simulink model "CombinedExperiment"  (R2020a)
settings: Solver=FixedStepAuto  StartTime=0.0  StopTime=tsim  FixedStep=baseRate  RelTol=1e-3  EnableMultiTasking=on
values from neighbouring files (symbols this model uses):
  baseRate = 1/10    (= 0.1)    [Run_Initializer.m]
  drop_states_BLACK = [ 0.6; 0.6; target_starting_angle]    [Run_Initializer.m]
  drop_states_BLUE = [ xLength/2+0.9; yLength/2+0.5; 0]    [Run_Initializer.m]
  drop_states_RED = [ xLength/2+0.6; yLength/2; pi]    [Run_Initializer.m]
  F_thrusters_BLACK = 0.25.*ones(8,1)    [Run_Initializer.m]
  F_thrusters_BLUE = 0.25.*ones(8,1)    [Run_Initializer.m]
  F_thrusters_RED = 0.25.*ones(8,1)    [Run_Initializer.m]
  home_states_BLACK = [ 0.6; 0.6; target_starting_angle]    [Run_Initializer.m]
  home_states_BLUE = [ xLength/2-0.9; yLength/2+0.5; 0]    [Run_Initializer.m]
  home_states_RED = [ xLength/2+0.6; yLength/2; pi]    [Run_Initializer.m]
  init_states_BLACK = [ 0.6; 0.6; target_starting_angle]    [Run_Initializer.m]
  init_states_BLUE = [ xLength/2+0.9; yLength/2+0.5; 0]    [Run_Initializer.m]
  init_states_RED = [ xLength/2+0.6; yLength/2; pi]    [Run_Initializer.m]
  Kd_tb = 0.4/5    (= 0.08)    [Run_Initializer.m]
  Kd_tblue = 0.4    [Run_Initializer.m]
  Kd_tr = 0.4    [Run_Initializer.m]
  Kd_xb = 5    [Run_Initializer.m]
  Kd_xblue = 5    [Run_Initializer.m]
  Kd_xr = 5    [Run_Initializer.m]
  Kd_yb = 5    [Run_Initializer.m]
  Kd_yblue = 5    [Run_Initializer.m]
  Kd_yr = 5    [Run_Initializer.m]
  Kp_tb = 0.1/5    (= 0.02)    [Run_Initializer.m]
  Kp_tblue = 0.1    [Run_Initializer.m]
  Kp_tr = 0.1    [Run_Initializer.m]
  Kp_xb = 2    [Run_Initializer.m]
  Kp_xblue = 2    [Run_Initializer.m]
  Kp_xr = 2    [Run_Initializer.m]
  Kp_yb = 2    [Run_Initializer.m]
  Kp_yblue = 2    [Run_Initializer.m]
  Kp_yr = 2    [Run_Initializer.m]
  noise_variance_BLACK = 0    [Run_Initializer.m]
  noise_variance_BLUE = 0    [Run_Initializer.m]
  noise_variance_RED = 0    [Run_Initializer.m]
  Phase0_End = Phase0_Duration    (= 8)    [Run_Initializer.m]
  Phase1_End = Phase0_Duration + Phase1_Duration    (= 13)    [Run_Initializer.m]
  Phase2_End = Phase0_Duration + Phase1_Duration +                                   Phase2_Duration    (= 38)    [Run_Initializer.m]
  Phase3_End = Phase0_Duration + Phase1_Duration +                                   Phase2_Duration + Phase3_Duration    (= 215)    [Run_Initializer.m]
  Phase3_SubPhase1_End = Phase2_End + Phase3_SubPhase1_Duration    (= 41)    [Run_Initializer.m]
  Phase3_SubPhase2_End = Phase2_End + Phase3_SubPhase1_Duration +                                   Phase3_SubPhase2_Duration    (= 42)    [Run_Initializer.m]
  Phase3_SubPhase3_End = Phase2_End + Phase3_SubPhase1_Duration +                                   Phase3_SubPhase2_Duration +                                  Phase3_SubPhase3_Duration    (= 72)    [Run_Initializer.m]
  Phase3_SubPhase4_End = Phase2_End + Phase3_SubPhase1_Duration +                                   Phase3_SubPhase2_Duration +                                  Phase3_SubPhase3_Duration +                                  Phase3_SubPhase4_Duration    [Run_Initializer.m]
  Phase4_End = Phase0_Duration + Phase1_Duration +                                   Phase2_Duration + Phase3_Duration +                                   Phase4_Duration    (= 235)    [Run_Initializer.m]
  Phase5_End = Phase0_Duration + Phase1_Duration +                                   Phase2_Duration + Phase3_Duration +                                   Phase4_Duration + Phase5_Duration    (= 240)    [Run_Initializer.m]
  serverRate = 1/5    (= 0.2)    [Run_Initializer.m]
  target_angular_velocity = 0.1    [Run_Initializer.m]
  thruster_dist2CG_BLACK = [83.42;-52.58;55.94;-60.05;54.08;-53.92;77.06;-55.94]    [Run_Initializer.m]
  thruster_dist2CG_BLUE = [83.42;-52.58;55.94;-60.05;54.08;-53.92;77.06;-55.94]    [Run_Initializer.m]
  thruster_dist2CG_RED = [49.92;-78.08;70.46;-63.54;81.08;-50.42;57.44;-75.96]    [Run_Initializer.m]
undefined symbols (not defined in the file or in its folder): DiscIntNeverNeededParam, platformSelection, simMode, WhoAmI
libraries: dspstat3 x18, dspsigops x12, raspberrypiBasiclib x10, embdlinuxlib x8, simulink x8, MainLibrary x6, mspfiltlib x3, dsparch4 x3, dspswit3 x2, sensehatlib x1
(part 5 of 10)

== system CombinedExperiment/Phase #3: Experiment/Change RED Behavior/Sub-Phase #3  ==
  note: ARM Control Law - RED
  note: PD Control Law - RED
  note: Additional Blocks
  note: Additional blocks are stored above. Note that to control attitude using the RW, simply replace RED_Tz with RED_Tz_RW.
  note: This section is reserved for any control law for the robotic manipulator.
  Action Port : ActionPort  ActionPortLabel=elseif( u1 < u4)
  1-D Lookup Table : Lookup_n-D  NumberOfTableDimensions=1  BreakpointsForDimension1=|  Table=|  InternalRulePriority=Speed  RndMeth=Simplest  InputSameDT=on
      BreakpointsForDimension1=|
      | [42
      | 42.01112133
      | 42.03727126
      | 42.07834039
      | 42.13428459
      | 42.20504754
      | 42.29055854
      | 42.39073228
      | 42.5054689
      | 42.63465399
      | 42.77815879
      | 42.93584024
      | 43.10754115
      | 43.29309037
      | 43.49230294
      | 43.70498028
      | 43.93091039
      | 44.16986804
      | 44.42161506
      | 44.68590048
      | 44.96246087
      | 45.25102053
      | 45.55129184
      | 45.86297547
      | 46.18576072
      | 46.51932585
      | 46.86333834
      | 47.21745527
      | 47.58132366
      | 47.95458079
      | 48.33685459
      | 48.727764
      | 49.12691936
      | 49.53392277
      | 49.94836853
      | 50.36984352
      | 50.79792758
      | 51.23219401
      | 51.67220991
      | 52.11753667
      | 52.56773038
      | 53.02234226
      | 53.48091917
      | 53.94300397
      | 54.40813605
      | 54.87585175
      | 55.34568486
      | 55.81716702
      | 56.28982825
      | 56.7631974
      | 57.2368026
      | 57.71017175
      | 58.18283298
      | 58.65431514
      | 59.12414825
      | 59.59186395
      | 60.05699603
      | 60.51908083
      | 60.97765774
      | 61.43226962
      | 61.88246333
      | 62.32779009
      | 62.76780599
      | 63.20207242
      | 63.63015648
      | 64.05163147
      | 64.46607723
      | 64.87308064
      | 65.272236
      | 65.66314541
      | 66.04541921
      | 66.41867634
      | 66.78254473
      | 67.13666166
      | 67.48067415
      | 67.81423928
      | 68.13702453
      | 68.44870816
      | 68.74897947
      | 69.03753913
      | 69.31409952
      | 69.57838494
      | 69.83013196
      | 70.06908961
      | 70.29501972
      | 70.50769706
      | 70.70690963
      | 70.89245885
      | 71.06415976
      | 71.22184121
      | 71.36534601
      | 71.4945311
      | 71.60926772
      | 71.70944146
      | 71.79495246
      | 71.86571541
      | 71.92165961
      | 71.96272874
      | 71.98887867
      | 72
      | ]
      Table=|
      | [1.570796327
      | 1.570792957
      | 1.570647694
      | 1.56961565
      | 1.567632601
      | 1.56219496
      | 1.557494298
      | 1.549269077
      | 1.544187815
      | 1.533149542
      | 1.522693414
      | 1.496131515
      | 1.446175572
      | 1.373291416
      | 1.270392573
      | 1.167493418
      | 1.052460989
      | 0.935207834
      | 0.807889258
      | 0.677163853
      | 0.538528963
      | 0.394913096
      | 0.249656169
      | 0.099916299
      | -0.053813644
      | -0.205103655
      | -0.380299244
      | -0.546735993
      | -0.717860815
      | -0.811444171
      | -0.923417052
      | -0.9559831
      | -0.833382367
      | -0.653115778
      | -0.440627342
      | -0.233135617
      | -0.016770488
      | 0.198541763
      | 0.420037648
      | 0.64133109
      | 0.8678487
      | 1.093144441
      | 1.326954733
      | 1.513077918
      | 1.568710242
      | 1.570730531
      | 1.567250769
      | 1.570752371
      | 1.57074092
      | 1.549011834
      | 1.401751602
      | 1.165146113
      | 1.0076873
      | 0.810904438
      | 0.65519077
      | 0.460795111
      | 0.26479445
      | 0.068785172
      | -0.154928236
      | -0.361424338
      | -0.588740331
      | -0.797757514
      | -1.025114417
      | -1.236311075
      | -1.435945334
      | -1.511406602
      | -1.466017975
      | -1.310813705
      | -1.105992736
      | -0.913718388
      | -0.722685301
      | -0.536202121
      | -0.354350457
      | -0.177037457
      | -0.005416103
      | 0.161859666
      | 0.322652337
      | 0.479244088
      | 0.627815916
      | 0.771700562
      | 0.909552257
      | 1.042365309
      | 1.164760086
      | 1.265366299
      | 1.329745445
      | 1.358265779
      | 1.355564401
      | 1.328554047
      | 1.279612684
      | 1.24723853
      | 1.197192467
      | 1.141005155
      | 1.106426692
      | 1.08119376
      | 1.067581158
      | 1.058578831
      | 1.055001377
      | 1.05322972
      | 1.052803704
      | 1.052721605
      | ]
  1-D Lookup Table1 : Lookup_n-D  NumberOfTableDimensions=1  BreakpointsForDimension1=|  Table=|  InternalRulePriority=Speed  RndMeth=Simplest  InputSameDT=on
      BreakpointsForDimension1=|
      | [42
      | 42.01112133
      | 42.03727126
      | 42.07834039
      | 42.13428459
      | 42.20504754
      | 42.29055854
      | 42.39073228
      | 42.5054689
      | 42.63465399
      | 42.77815879
      | 42.93584024
      | 43.10754115
      | 43.29309037
      | 43.49230294
      | 43.70498028
      | 43.93091039
      | 44.16986804
      | 44.42161506
      | 44.68590048
      | 44.96246087
      | 45.25102053
      | 45.55129184
      | 45.86297547
      | 46.18576072
      | 46.51932585
      | 46.86333834
      | 47.21745527
      | 47.58132366
      | 47.95458079
      | 48.33685459
      | 48.727764
      | 49.12691936
      | 49.53392277
      | 49.94836853
      | 50.36984352
      | 50.79792758
      | 51.23219401
      | 51.67220991
      | 52.11753667
      | 52.56773038
      | 53.02234226
      | 53.48091917
      | 53.94300397
      | 54.40813605
      | 54.87585175
      | 55.34568486
      | 55.81716702
      | 56.28982825
      | 56.7631974
      | 57.2368026
      | 57.71017175
      | 58.18283298
      | 58.65431514
      | 59.12414825
      | 59.59186395
      | 60.05699603
      | 60.51908083
      | 60.97765774
      | 61.43226962
      | 61.88246333
      | 62.32779009
      | 62.76780599
      | 63.20207242
      | 63.63015648
      | 64.05163147
      | 64.46607723
      | 64.87308064
      | 65.272236
      | 65.66314541
      | 66.04541921
      | 66.41867634
      | 66.78254473
      | 67.13666166
      | 67.48067415
      | 67.81423928
      | 68.13702453
      | 68.44870816
      | 68.74897947
      | 69.03753913
      | 69.31409952
      | 69.57838494
      | 69.83013196
      | 70.06908961
      | 70.29501972
      | 70.50769706
      | 70.70690963
      | 70.89245885
      | 71.06415976
      | 71.22184121
      | 71.36534601
      | 71.4945311
      | 71.60926772
      | 71.70944146
      | 71.79495246
      | 71.86571541
      | 71.92165961
      | 71.96272874
      | 71.98887867
      | 72
      | ]
      Table=|
      | [1.57079632679490
      | 1.57079662136271
      | 1.57035858393418
      | 1.56955473957150
      | 1.56795883023701
      | 1.56855196252543
      | 1.56956191136717
      | 1.57072970527338
      | 1.57079005485722
      | 1.56948791223666
      | 1.55119006552306
      | 1.55836585845583
      | 1.57077777185491
      | 1.57077149370545
      | 1.57076310797240
      | 1.57036928804412
      | 1.57074947684855
      | 1.56898331366692
      | 1.57073740451593
      | 1.56257826917437
      | 1.57072974696569
      | 1.56230742665956
      | 1.57073312881541
      | 1.56360724537446
      | 1.57075185491036
      | 1.56920954766940
      | 1.57077382899638
      | 1.54477346684241
      | 1.38400507014983
      | 1.23109269186081
      | 1.02321737126326
      | 0.866665055111140
      | 0.663320579242585
      | 0.523334911886864
      | 0.348534652658928
      | 0.228481728516264
      | 0.156644623807384
      | 0.0854385589397119
      | 0.0684187356026291
      | -0.0143597952556130
      | -0.0517524216410004
      | -0.0928804549026143
      | -0.215704480084781
      | -0.422252680325216
      | -0.607845118006062
      | -0.846263996013364
      | -1.04958098308095
      | -1.27739473865326
      | -1.42310649047080
      | -1.57075277736191
      | -1.57072459354704
      | -1.57072993276777
      | -1.54331811766860
      | -1.57073414073308
      | -1.55931623516956
      | -1.57073842553777
      | -1.57072399077284
      | -1.57072720156105
      | -1.57071264380253
      | -1.56934197452670
      | -1.57070564382063
      | -1.56141817042798
      | -1.57070830688086
      | -1.49469854852628
      | -1.31259934378585
      | -1.11020895684375
      | -0.916078821647610
      | -0.731793274192232
      | -0.573229556030265
      | -0.475634259727501
      | -0.252113034776861
      | -0.175932768714599
      | -0.117451385657779
      | -0.113075584941122
      | -0.108548532723191
      | -0.120323450723243
      | -0.116071199535664
      | -0.122092030089114
      | -0.179069682787195
      | -0.187679506880811
      | -0.283142131452161
      | -0.409036068532655
      | -0.536944980678811
      | -0.655297933993903
      | -0.768540738868273
      | -0.875433002578302
      | -0.973536605110186
      | -1.06911393555782
      | -1.14791786909907
      | -1.22902449271238
      | -1.27006052589809
      | -1.28669314276116
      | -1.31617501989999
      | -1.33099075176741
      | -1.34662299508091
      | -1.35249457213426
      | -1.35797341773929
      | -1.35939252934314
      | -1.35990006404006
      | -1.35985448160842]
  1-D Lookup Table2 : Lookup_n-D  NumberOfTableDimensions=1  BreakpointsForDimension1=|  Table=|  InternalRulePriority=Speed  RndMeth=Simplest  InputSameDT=on
      BreakpointsForDimension1=|
      | [42
      | 42.01112133
      | 42.03727126
      | 42.07834039
      | 42.13428459
      | 42.20504754
      | 42.29055854
      | 42.39073228
      | 42.5054689
      | 42.63465399
      | 42.77815879
      | 42.93584024
      | 43.10754115
      | 43.29309037
      | 43.49230294
      | 43.70498028
      | 43.93091039
      | 44.16986804
      | 44.42161506
      | 44.68590048
      | 44.96246087
      | 45.25102053
      | 45.55129184
      | 45.86297547
      | 46.18576072
      | 46.51932585
      | 46.86333834
      | 47.21745527
      | 47.58132366
      | 47.95458079
      | 48.33685459
      | 48.727764
      | 49.12691936
      | 49.53392277
      | 49.94836853
      | 50.36984352
      | 50.79792758
      | 51.23219401
      | 51.67220991
      | 52.11753667
      | 52.56773038
      | 53.02234226
      | 53.48091917
      | 53.94300397
      | 54.40813605
      | 54.87585175
      | 55.34568486
      | 55.81716702
      | 56.28982825
      | 56.7631974
      | 57.2368026
      | 57.71017175
      | 58.18283298
      | 58.65431514
      | 59.12414825
      | 59.59186395
      | 60.05699603
      | 60.51908083
      | 60.97765774
      | 61.43226962
      | 61.88246333
      | 62.32779009
      | 62.76780599
      | 63.20207242
      | 63.63015648
      | 64.05163147
      | 64.46607723
      | 64.87308064
      | 65.272236
      | 65.66314541
      | 66.04541921
      | 66.41867634
      | 66.78254473
      | 67.13666166
      | 67.48067415
      | 67.81423928
      | 68.13702453
      | 68.44870816
      | 68.74897947
      | 69.03753913
      | 69.31409952
      | 69.57838494
      | 69.83013196
      | 70.06908961
      | 70.29501972
      | 70.50769706
      | 70.70690963
      | 70.89245885
      | 71.06415976
      | 71.22184121
      | 71.36534601
      | 71.4945311
      | 71.60926772
      | 71.70944146
      | 71.79495246
      | 71.86571541
      | 71.92165961
      | 71.96272874
      | 71.98887867
      | 72
      | ]
      Table=|
      | [-1.10360555189321e-17
      | -0.000682555954124297
      | -0.000504375242443253
      | 0.00336297359381415
      | 0.0137095670724727
      | 0.0252677971790659
      | 0.0446557220510096
      | 0.0672113326003172
      | 0.0999781977666613
      | 0.137287456967193
      | 0.189071248486376
      | 0.272294508037825
      | 0.355665679231944
      | 0.446845913729827
      | 0.544137284526667
      | 0.639346413276106
      | 0.732541458867562
      | 0.808938354869002
      | 0.855848674103189
      | 0.891616122311551
      | 0.876064789878543
      | 0.835218274860764
      | 0.735847487773707
      | 0.623237833236767
      | 0.450912596118759
      | 0.313068707480842
      | 0.118982751928026
      | -0.0346963999777990
      | -0.244244268013732
      | -0.386045753956551
      | -0.607135995230889
      | -0.645065479955685
      | -0.658232101032023
      | -0.707283001569499
      | -0.727739337943063
      | -0.773334139757485
      | -0.790813868197939
      | -0.829315581367480
      | -0.831591865361474
      | -0.895741116707505
      | -0.917692198886409
      | -0.966835773186509
      | -1.05732301030663
      | -1.15418729750044
      | -1.28905944926691
      | -1.41505461173534
      | -1.40486598987903
      | -1.38850533888304
      | -1.31148648974968
      | -1.22739644537344
      | -1.09679708257291
      | -1.01375741649069
      | -0.900389419892854
      | -0.817697106109663
      | -0.706296706872995
      | -0.627649901158471
      | -0.522783214749143
      | -0.449254069405809
      | -0.350308226521183
      | -0.271181857633944
      | -0.185730374564875
      | -0.134238582279295
      | -0.0589333568892688
      | -0.0193632216828676
      | 0.0500980441953301
      | 0.0783818433368992
      | 0.203392718385905
      | 0.287418813233287
      | 0.286916152215522
      | 0.228277773431529
      | 0.205391483508272
      | 0.153166933412198
      | 4.01249706205260e-05
      | -0.106583281044124
      | -0.214939176631723
      | -0.275105513577021
      | -0.328996825397653
      | -0.353637536054736
      | -0.366278937268333
      | -0.349072653017436
      | -0.324125317636826
      | -0.291582405014021
      | -0.240949835499918
      | -0.195848531903513
      | -0.143488080387155
      | -0.0988801304986467
      | -0.0443831356850743
      | 0.00807376276159867
      | 0.0766461923527033
      | 0.116804310925055
      | 0.159885004199221
      | 0.212747759359235
      | 0.240304582731963
      | 0.265011768867661
      | 0.280740585503698
      | 0.294154580752225
      | 0.300980006322197
      | 0.305531467486406
      | 0.306822115333088
      | 0.307132876918720]
  Constant{,1,4..6} (5 alike) : Constant  Value=0
  Data Store Read : DataStoreRead  DataStoreName=Univ_Time
  Data Store Write : DataStoreWrite  DataStoreName=RED_Tz_Shoulder
  Data Store Write1 : DataStoreWrite  DataStoreName=RED_Tz_Elbow
  Data Store Write2 : DataStoreWrite  DataStoreName=RED_Tz_Wrist
  Data Store Write3 : DataStoreWrite  DataStoreName=Float_State
  From Workspace : FromWorkspace  Commented=on  VariableName=Pos_J1  SampleTime=-1
  From Workspace1 : FromWorkspace  Commented=on  VariableName=Pos_J2  SampleTime=-1
  From Workspace2 : FromWorkspace  Commented=on  VariableName=Pos_J3  SampleTime=-1
  Puck State : Constant
  RED_Fx : DataStoreWrite  DataStoreName=RED_Fx
  RED_Fy : DataStoreWrite  DataStoreName=RED_Fy
  RED_Tz : DataStoreWrite  DataStoreName=RED_Tz
  RED_Tz_RW : DataStoreWrite  DataStoreName=RED_Tz_RW
  Send Position Commands to Manipulator : MainLibrary/Dynamixel Functions/Send Position Commands to Manipulator  Commented=on
      settings: SourceProductName=SPOT Custom Library
  Send Position Commands to Manipulator1 : MainLibrary/Dynamixel Functions/Send Position Commands to Manipulator
      settings: SourceProductName=SPOT Custom Library
  wires:
  Constant1/1 -> RED_Tz_RW/1
  Constant6/1 -> Data Store Write2/1
  Constant4/1 -> Data Store Write/1
  Constant5/1 -> Data Store Write1/1
  Constant/1 -> RED_Tz/1, RED_Fx/1, RED_Fy/1
  Puck State/1 -> Data Store Write3/1
  From Workspace2/1 -> Send Position Commands to Manipulator/3
  From Workspace1/1 -> Send Position Commands to Manipulator/2
  From Workspace/1 -> Send Position Commands to Manipulator/1
  1-D Lookup Table2/1 -> Send Position Commands to Manipulator1/3
  Data Store Read/1 -> 1-D Lookup Table2/1, 1-D Lookup Table1/1, 1-D Lookup Table/1
  1-D Lookup Table1/1 -> Send Position Commands to Manipulator1/2
  1-D Lookup Table/1 -> Send Position Commands to Manipulator1/1

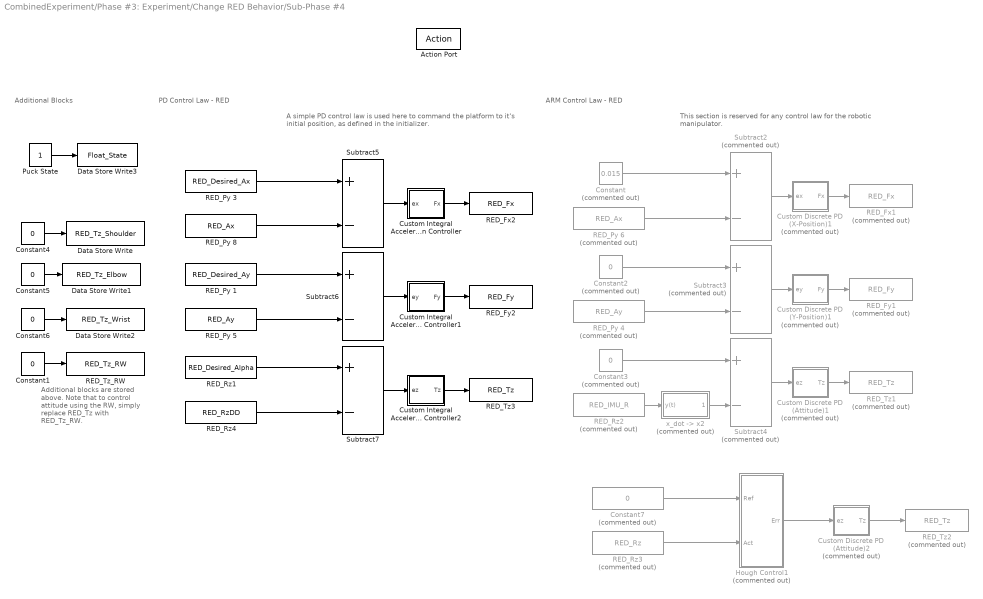
== system CombinedExperiment/Phase #3: Experiment/Change RED Behavior/Sub-Phase #4 ==
  note: ARM Control Law - RED
  note: PD Control Law - RED
  note: Additional Blocks
  note: Additional blocks are stored above. Note that to control attitude using the RW, simply replace RED_Tz with RED_Tz_RW.
  note: A simple PD control law is used here to command the platform to it's initial position, as defined in the initializer.
  note: This section is reserved for any control law for the robotic manipulator.
  Action Port : ActionPort  ActionPortLabel=elseif( u1 < u5)
  Constant : Constant  Commented=on  Value=0.015
  Constant{1,4..6} (4 alike) : Constant  Value=0
  Constant2 : Constant  Commented=on  Value=0
  Constant3 : Constant  Commented=on  Value=0
  Constant7 : Constant  Commented=on  Value=0
  Custom Discrete PD (Attitude)1 : Subsystem  Commented=on
  Custom Discrete PD (Attitude)2 : Subsystem  Commented=on
  Custom Discrete PD (X-Position)1 : Subsystem  Commented=on
  Custom Discrete PD (Y-Position)1 : Subsystem  Commented=on
  Custom Integral Acceleration Controller : Subsystem
  Custom Integral Acceleration Controller1 : Subsystem
  Custom Integral Acceleration Controller2 : Subsystem
  Data Store Write : DataStoreWrite  DataStoreName=RED_Tz_Shoulder
  Data Store Write1 : DataStoreWrite  DataStoreName=RED_Tz_Elbow
  Data Store Write2 : DataStoreWrite  DataStoreName=RED_Tz_Wrist
  Data Store Write3 : DataStoreWrite  DataStoreName=Float_State
  Hough Control1 : Subsystem  Commented=on
  Puck State : Constant
  RED_Fx1 : DataStoreWrite  Commented=on  DataStoreName=RED_Fx
  RED_Fx2 : DataStoreWrite  DataStoreName=RED_Fx
  RED_Fy1 : DataStoreWrite  Commented=on  DataStoreName=RED_Fy
  RED_Fy2 : DataStoreWrite  DataStoreName=RED_Fy
  RED_Py 1 : DataStoreRead  DataStoreName=RED_Desired_Ay
  RED_Py 3 : DataStoreRead  DataStoreName=RED_Desired_Ax
  RED_Py 4 : DataStoreRead  Commented=on  DataStoreName=RED_Ay
  RED_Py 5 : DataStoreRead  DataStoreName=RED_Ay
  RED_Py 6 : DataStoreRead  Commented=on  DataStoreName=RED_Ax
  RED_Py 8 : DataStoreRead  DataStoreName=RED_Ax
  RED_Rz1 : DataStoreRead  DataStoreName=RED_Desired_Alpha
  RED_Rz2 : DataStoreRead  Commented=on  DataStoreName=RED_IMU_R
  RED_Rz3 : DataStoreRead  Commented=on  DataStoreName=RED_Rz
  RED_Rz4 : DataStoreRead  DataStoreName=RED_RzDD
  RED_Tz1 : DataStoreWrite  Commented=on  DataStoreName=RED_Tz
  RED_Tz2 : DataStoreWrite  Commented=on  DataStoreName=RED_Tz
  RED_Tz3 : DataStoreWrite  DataStoreName=RED_Tz
  RED_Tz_RW : DataStoreWrite  DataStoreName=RED_Tz_RW
  Subtract2 : Sum  Commented=on  Inputs=+-
  Subtract3 : Sum  Commented=on  Inputs=+-
  Subtract4 : Sum  Commented=on  Inputs=+-
  Subtract5 : Sum  Inputs=+-
  Subtract6 : Sum  Inputs=+-
  Subtract7 : Sum  Inputs=+-
  "x_dot -> x2" : Subsystem  Commented=on
  wires:
  Constant1/1 -> RED_Tz_RW/1
  Constant6/1 -> Data Store Write2/1
  Constant4/1 -> Data Store Write/1
  Constant5/1 -> Data Store Write1/1
  Puck State/1 -> Data Store Write3/1
  Constant2/1 -> Subtract3/1
  "x_dot -> x2"/1(dy(t)/dt) -> Subtract4/2
  Subtract3/1 -> Custom Discrete PD (Y-Position)1/1(ey)
  Constant3/1 -> Subtract4/1
  RED_Py 4/1 -> Subtract3/2
  RED_Rz2/1 -> "x_dot -> x2"/1(y(t))
  Custom Discrete PD (Attitude)1/1(Tz) -> RED_Tz1/1
  RED_Py 6/1 -> Subtract2/2
  Subtract2/1 -> Custom Discrete PD (X-Position)1/1(ex)
  Custom Discrete PD (X-Position)1/1(Fx) -> RED_Fx1/1
  Subtract4/1 -> Custom Discrete PD (Attitude)1/1(ez)
  Constant/1 -> Subtract2/1
  Custom Discrete PD (Y-Position)1/1(Fy) -> RED_Fy1/1
  Hough Control1/1(Err) -> Custom Discrete PD (Attitude)2/1(ez)
  Constant7/1 -> Hough Control1/1(Ref)
  RED_Rz3/1 -> Hough Control1/2(Act)
  Custom Discrete PD (Attitude)2/1(Tz) -> RED_Tz2/1
  Subtract6/1 -> Custom Integral Acceleration Controller1/1(ey)
  Subtract5/1 -> Custom Integral Acceleration Controller/1(ex)
  RED_Py 8/1 -> Subtract5/2
  RED_Rz4/1 -> Subtract7/2
  Subtract7/1 -> Custom Integral Acceleration Controller2/1(ez)
  RED_Py 5/1 -> Subtract6/2
  Custom Integral Acceleration Controller2/1(Tz) -> RED_Tz3/1
  Custom Integral Acceleration Controller1/1(Fy) -> RED_Fy2/1
  Custom Integral Acceleration Controller/1(Fx) -> RED_Fx2/1
  RED_Py 3/1 -> Subtract5/1
  RED_Py 1/1 -> Subtract6/1
  RED_Rz1/1 -> Subtract7/1

== system CombinedExperiment/Phase #3: Experiment/Change RED Behavior/Subsystem ==
  Universal_Time : DataStoreRead  DataStoreName=Univ_Time
  Time : Outport  VectorParamsAs1DForOutWhenUnconnected=off
  wires:
  Universal_Time/1 -> Time/1

== system CombinedExperiment/Phase #4: Return Home/Change BLACK Behavior/Custom Discrete PD (Attitude) ==
  ez : Inport
  Sum3 : Sum
  kd_tb : Gain  Gain=Kd_tb
  kp_tb : Gain  Gain=Kp_tb
  "x_dot -> x1" : Subsystem
  Tz : Outport  VectorParamsAs1DForOutWhenUnconnected=off
  wires:
  kd_tb/1 -> Sum3/1
  Sum3/1 -> Tz/1
  kp_tb/1 -> Sum3/2
  "x_dot -> x1"/1(dy(t)/dt) -> kd_tb/1
  ez/1 -> "x_dot -> x1"/1(y(t)), kp_tb/1

== system CombinedExperiment/Phase #4: Return Home/Change BLACK Behavior/Custom Discrete PD (X-Position) ==
  ex : Inport
  Sum3 : Sum
  kd_xb : Gain  Gain=Kd_xb
  kp_xb : Gain  Gain=Kp_xb
  "x_dot -> x1" : Subsystem
  Fx : Outport  VectorParamsAs1DForOutWhenUnconnected=off
  wires:
  kd_xb/1 -> Sum3/1
  ex/1 -> "x_dot -> x1"/1(y(t)), kp_xb/1
  kp_xb/1 -> Sum3/2
  "x_dot -> x1"/1(dy(t)/dt) -> kd_xb/1
  Sum3/1 -> Fx/1

== system CombinedExperiment/Phase #4: Return Home/Change BLACK Behavior/Custom Discrete PD (Y-Position) ==
  ey : Inport
  Sum3 : Sum
  kd_yb : Gain  Gain=Kd_yb
  kp_yb : Gain  Gain=Kp_yb
  "x_dot -> x1" : Subsystem
  Fy : Outport  VectorParamsAs1DForOutWhenUnconnected=off
  wires:
  kd_yb/1 -> Sum3/1
  Sum3/1 -> Fy/1
  kp_yb/1 -> Sum3/2
  "x_dot -> x1"/1(dy(t)/dt) -> kd_yb/1
  ey/1 -> "x_dot -> x1"/1(y(t)), kp_yb/1

== system CombinedExperiment/Phase #4: Return Home/Change BLACK Behavior/Hough Control ==
  Ref : Inport
  Act : Inport  Port=2
  MATLAB Function2 : MATLAB Function  TreatAsAtomicUnit=on
  MATLAB Function3 : MATLAB Function  TreatAsAtomicUnit=on
  MATLAB Function4 : MATLAB Function  TreatAsAtomicUnit=on
  Subtract2 : Sum  Inputs=+-
  Err : Outport  VectorParamsAs1DForOutWhenUnconnected=off
  wires:
  MATLAB Function4/1(e_out) -> Err/1
  MATLAB Function2/1(Oy) -> MATLAB Function4/1(Oy)
  Subtract2/1 -> MATLAB Function4/2(e_in)
  MATLAB Function2/2(Ox) -> Subtract2/1
  Act/1 -> MATLAB Function3/1(z)
  Ref/1 -> MATLAB Function2/1(z)
  MATLAB Function3/1(Ox) -> Subtract2/2

== system CombinedExperiment/Phase #4: Return Home/Change BLUE Behavior/Custom Discrete PD (Attitude) ==
  ez : Inport
  Sum3 : Sum
  kd_tb : Gain  Gain=Kd_tblue
  kp_tb : Gain  Gain=Kp_tblue
  "x_dot -> x1" : Subsystem
  Tz : Outport  VectorParamsAs1DForOutWhenUnconnected=off
  wires:
  kd_tb/1 -> Sum3/1
  Sum3/1 -> Tz/1
  kp_tb/1 -> Sum3/2
  "x_dot -> x1"/1(dy(t)/dt) -> kd_tb/1
  ez/1 -> "x_dot -> x1"/1(y(t)), kp_tb/1

== system CombinedExperiment/Phase #4: Return Home/Change BLUE Behavior/Custom Discrete PD (X-Position) ==
  ex : Inport
  Sum3 : Sum
  kd_xb : Gain  Gain=Kd_xblue
  kp_xb : Gain  Gain=Kp_xblue
  "x_dot -> x1" : Subsystem
  Fx : Outport  VectorParamsAs1DForOutWhenUnconnected=off
  wires:
  kd_xb/1 -> Sum3/1
  ex/1 -> "x_dot -> x1"/1(y(t)), kp_xb/1
  kp_xb/1 -> Sum3/2
  "x_dot -> x1"/1(dy(t)/dt) -> kd_xb/1
  Sum3/1 -> Fx/1

== system CombinedExperiment/Phase #4: Return Home/Change BLUE Behavior/Custom Discrete PD (Y-Position) ==
  ey : Inport
  Sum3 : Sum
  kd_yb : Gain  Gain=Kd_yblue
  kp_yb : Gain  Gain=Kp_yblue
  "x_dot -> x1" : Subsystem
  Fy : Outport  VectorParamsAs1DForOutWhenUnconnected=off
  wires:
  kd_yb/1 -> Sum3/1
  Sum3/1 -> Fy/1
  kp_yb/1 -> Sum3/2
  "x_dot -> x1"/1(dy(t)/dt) -> kd_yb/1
  ey/1 -> "x_dot -> x1"/1(y(t)), kp_yb/1

== system CombinedExperiment/Phase #4: Return Home/Change BLUE Behavior/Hough Control ==
  Ref : Inport
  Act : Inport  Port=2
  MATLAB Function2 : MATLAB Function  TreatAsAtomicUnit=on
  MATLAB Function3 : MATLAB Function  TreatAsAtomicUnit=on
  MATLAB Function4 : MATLAB Function  TreatAsAtomicUnit=on
  Subtract2 : Sum  Inputs=+-
  Err : Outport  VectorParamsAs1DForOutWhenUnconnected=off
  wires:
  MATLAB Function4/1(e_out) -> Err/1
  MATLAB Function2/1(Oy) -> MATLAB Function4/1(Oy)
  Subtract2/1 -> MATLAB Function4/2(e_in)
  MATLAB Function2/2(Ox) -> Subtract2/1
  Act/1 -> MATLAB Function3/1(z)
  Ref/1 -> MATLAB Function2/1(z)
  MATLAB Function3/1(Ox) -> Subtract2/2

== system CombinedExperiment/Phase #4: Return Home/Change RED Behavior/Custom Discrete PD (Attitude) ==
  ez : Inport
  Sum3 : Sum
  kd_tr : Gain  Gain=Kd_tr
  kp_tr : Gain  Gain=Kp_tr
  "x_dot -> x1" : Subsystem
  Tz : Outport  VectorParamsAs1DForOutWhenUnconnected=off
  wires:
  kd_tr/1 -> Sum3/1
  Sum3/1 -> Tz/1
  kp_tr/1 -> Sum3/2
  "x_dot -> x1"/1(dy(t)/dt) -> kd_tr/1
  ez/1 -> "x_dot -> x1"/1(y(t)), kp_tr/1

== system CombinedExperiment/Phase #4: Return Home/Change RED Behavior/Custom Discrete PD (X-Position) ==
  ex : Inport
  Sum3 : Sum
  kd_xr : Gain  Gain=Kd_xr
  kp_xr : Gain  Gain=Kp_xr
  "x_dot -> x1" : Subsystem
  Fx : Outport  VectorParamsAs1DForOutWhenUnconnected=off
  wires:
  kd_xr/1 -> Sum3/1
  ex/1 -> "x_dot -> x1"/1(y(t)), kp_xr/1
  kp_xr/1 -> Sum3/2
  "x_dot -> x1"/1(dy(t)/dt) -> kd_xr/1
  Sum3/1 -> Fx/1

== system CombinedExperiment/Phase #4: Return Home/Change RED Behavior/Custom Discrete PD (Y-Position) ==
  ey : Inport
  Sum3 : Sum
  kd_yr : Gain  Gain=Kd_yr
  kp_yr : Gain  Gain=Kp_yr
  "x_dot -> x1" : Subsystem
  Fy : Outport  VectorParamsAs1DForOutWhenUnconnected=off
  wires:
  kd_yr/1 -> Sum3/1
  Sum3/1 -> Fy/1
  kp_yr/1 -> Sum3/2
  "x_dot -> x1"/1(dy(t)/dt) -> kd_yr/1
  ey/1 -> "x_dot -> x1"/1(y(t)), kp_yr/1

== system CombinedExperiment/Phase #4: Return Home/Change RED Behavior/Hough Control ==
  Ref : Inport
  Act : Inport  Port=2
  MATLAB Function2 : MATLAB Function  TreatAsAtomicUnit=on
  MATLAB Function3 : MATLAB Function  TreatAsAtomicUnit=on
  MATLAB Function4 : MATLAB Function  TreatAsAtomicUnit=on
  Subtract2 : Sum  Inputs=+-
  Err : Outport  VectorParamsAs1DForOutWhenUnconnected=off
  wires:
  MATLAB Function4/1(e_out) -> Err/1
  MATLAB Function2/1(Oy) -> MATLAB Function4/1(Oy)
  Subtract2/1 -> MATLAB Function4/2(e_in)
  MATLAB Function2/2(Ox) -> Subtract2/1
  Act/1 -> MATLAB Function3/1(z)
  Ref/1 -> MATLAB Function2/1(z)
  MATLAB Function3/1(Ox) -> Subtract2/2

== system CombinedExperiment/Phase #5: Hold Home/Change BLACK Behavior/Custom Discrete PD (Attitude) ==
  ez : Inport
  Sum3 : Sum
  kd_tb : Gain  Gain=Kd_tb
  kp_tb : Gain  Gain=Kp_tb
  "x_dot -> x1" : Subsystem
  Tz : Outport  VectorParamsAs1DForOutWhenUnconnected=off
  wires:
  kd_tb/1 -> Sum3/1
  Sum3/1 -> Tz/1
  kp_tb/1 -> Sum3/2
  "x_dot -> x1"/1(dy(t)/dt) -> kd_tb/1
  ez/1 -> "x_dot -> x1"/1(y(t)), kp_tb/1

== system CombinedExperiment/Phase #5: Hold Home/Change BLACK Behavior/Custom Discrete PD (X-Position) ==
  ex : Inport
  Sum3 : Sum
  kd_xb : Gain  Gain=Kd_xb
  kp_xb : Gain  Gain=Kp_xb
  "x_dot -> x1" : Subsystem
  Fx : Outport  VectorParamsAs1DForOutWhenUnconnected=off
  wires:
  kd_xb/1 -> Sum3/1
  ex/1 -> "x_dot -> x1"/1(y(t)), kp_xb/1
  kp_xb/1 -> Sum3/2
  "x_dot -> x1"/1(dy(t)/dt) -> kd_xb/1
  Sum3/1 -> Fx/1

== system CombinedExperiment/Phase #5: Hold Home/Change BLACK Behavior/Custom Discrete PD (Y-Position) ==
  ey : Inport
  Sum3 : Sum
  kd_yb : Gain  Gain=Kd_yb
  kp_yb : Gain  Gain=Kp_yb
  "x_dot -> x1" : Subsystem
  Fy : Outport  VectorParamsAs1DForOutWhenUnconnected=off
  wires:
  kd_yb/1 -> Sum3/1
  Sum3/1 -> Fy/1
  kp_yb/1 -> Sum3/2
  "x_dot -> x1"/1(dy(t)/dt) -> kd_yb/1
  ey/1 -> "x_dot -> x1"/1(y(t)), kp_yb/1

== system CombinedExperiment/Phase #5: Hold Home/Change BLACK Behavior/Hough Control ==
  Ref : Inport
  Act : Inport  Port=2
  MATLAB Function2 : MATLAB Function  TreatAsAtomicUnit=on
  MATLAB Function3 : MATLAB Function  TreatAsAtomicUnit=on
  MATLAB Function4 : MATLAB Function  TreatAsAtomicUnit=on
  Subtract2 : Sum  Inputs=+-
  Err : Outport  VectorParamsAs1DForOutWhenUnconnected=off
  wires:
  MATLAB Function4/1(e_out) -> Err/1
  MATLAB Function2/1(Oy) -> MATLAB Function4/1(Oy)
  Subtract2/1 -> MATLAB Function4/2(e_in)
  MATLAB Function2/2(Ox) -> Subtract2/1
  Act/1 -> MATLAB Function3/1(z)
  Ref/1 -> MATLAB Function2/1(z)
  MATLAB Function3/1(Ox) -> Subtract2/2

== system CombinedExperiment/Phase #5: Hold Home/Change BLUE Behavior/Custom Discrete PD (Attitude) ==
  ez : Inport
  Sum3 : Sum
  kd_tb : Gain  Gain=Kd_tblue
  kp_tb : Gain  Gain=Kp_tblue
  "x_dot -> x1" : Subsystem
  Tz : Outport  VectorParamsAs1DForOutWhenUnconnected=off
  wires:
  kd_tb/1 -> Sum3/1
  Sum3/1 -> Tz/1
  kp_tb/1 -> Sum3/2
  "x_dot -> x1"/1(dy(t)/dt) -> kd_tb/1
  ez/1 -> "x_dot -> x1"/1(y(t)), kp_tb/1

== system CombinedExperiment/Phase #5: Hold Home/Change BLUE Behavior/Custom Discrete PD (X-Position) ==
  ex : Inport
  Sum3 : Sum
  kd_xb : Gain  Gain=Kd_xblue
  kp_xb : Gain  Gain=Kp_xblue
  "x_dot -> x1" : Subsystem
  Fx : Outport  VectorParamsAs1DForOutWhenUnconnected=off
  wires:
  kd_xb/1 -> Sum3/1
  ex/1 -> "x_dot -> x1"/1(y(t)), kp_xb/1
  kp_xb/1 -> Sum3/2
  "x_dot -> x1"/1(dy(t)/dt) -> kd_xb/1
  Sum3/1 -> Fx/1

== system CombinedExperiment/Phase #5: Hold Home/Change BLUE Behavior/Custom Discrete PD (Y-Position) ==
  ey : Inport
  Sum3 : Sum
  kd_yb : Gain  Gain=Kd_yblue
  kp_yb : Gain  Gain=Kp_yblue
  "x_dot -> x1" : Subsystem
  Fy : Outport  VectorParamsAs1DForOutWhenUnconnected=off
  wires:
  kd_yb/1 -> Sum3/1
  Sum3/1 -> Fy/1
  kp_yb/1 -> Sum3/2
  "x_dot -> x1"/1(dy(t)/dt) -> kd_yb/1
  ey/1 -> "x_dot -> x1"/1(y(t)), kp_yb/1

== system CombinedExperiment/Phase #5: Hold Home/Change BLUE Behavior/Hough Control ==
  Ref : Inport
  Act : Inport  Port=2
  MATLAB Function2 : MATLAB Function  TreatAsAtomicUnit=on
  MATLAB Function3 : MATLAB Function  TreatAsAtomicUnit=on
  MATLAB Function4 : MATLAB Function  TreatAsAtomicUnit=on
  Subtract2 : Sum  Inputs=+-
  Err : Outport  VectorParamsAs1DForOutWhenUnconnected=off
  wires:
  MATLAB Function4/1(e_out) -> Err/1
  MATLAB Function2/1(Oy) -> MATLAB Function4/1(Oy)
  Subtract2/1 -> MATLAB Function4/2(e_in)
  MATLAB Function2/2(Ox) -> Subtract2/1
  Act/1 -> MATLAB Function3/1(z)
  Ref/1 -> MATLAB Function2/1(z)
  MATLAB Function3/1(Ox) -> Subtract2/2

== system CombinedExperiment/Phase #5: Hold Home/Change RED Behavior/Custom Discrete PD (Attitude) ==
  ez : Inport
  Sum3 : Sum
  kd_tr : Gain  Gain=Kd_tr
  kp_tr : Gain  Gain=Kp_tr
  "x_dot -> x1" : Subsystem
  Tz : Outport  VectorParamsAs1DForOutWhenUnconnected=off
  wires:
  kd_tr/1 -> Sum3/1
  Sum3/1 -> Tz/1
  kp_tr/1 -> Sum3/2
  "x_dot -> x1"/1(dy(t)/dt) -> kd_tr/1
  ez/1 -> "x_dot -> x1"/1(y(t)), kp_tr/1

== system CombinedExperiment/Phase #5: Hold Home/Change RED Behavior/Custom Discrete PD (X-Position) ==
  ex : Inport
  Sum3 : Sum
  kd_xr : Gain  Gain=Kd_xr
  kp_xr : Gain  Gain=Kp_xr
  "x_dot -> x1" : Subsystem
  Fx : Outport  VectorParamsAs1DForOutWhenUnconnected=off
  wires:
  kd_xr/1 -> Sum3/1
  ex/1 -> "x_dot -> x1"/1(y(t)), kp_xr/1
  kp_xr/1 -> Sum3/2
  "x_dot -> x1"/1(dy(t)/dt) -> kd_xr/1
  Sum3/1 -> Fx/1

== system CombinedExperiment/Phase #5: Hold Home/Change RED Behavior/Custom Discrete PD (Y-Position) ==
  ey : Inport
  Sum3 : Sum
  kd_yr : Gain  Gain=Kd_yr
  kp_yr : Gain  Gain=Kp_yr
  "x_dot -> x1" : Subsystem
  Fy : Outport  VectorParamsAs1DForOutWhenUnconnected=off
  wires:
  kd_yr/1 -> Sum3/1
  Sum3/1 -> Fy/1
  kp_yr/1 -> Sum3/2
  "x_dot -> x1"/1(dy(t)/dt) -> kd_yr/1
  ey/1 -> "x_dot -> x1"/1(y(t)), kp_yr/1

== system CombinedExperiment/Phase #5: Hold Home/Change RED Behavior/Hough Control ==
  Ref : Inport
  Act : Inport  Port=2
  MATLAB Function2 : MATLAB Function  TreatAsAtomicUnit=on
  MATLAB Function3 : MATLAB Function  TreatAsAtomicUnit=on
  MATLAB Function4 : MATLAB Function  TreatAsAtomicUnit=on
  Subtract2 : Sum  Inputs=+-
  Err : Outport  VectorParamsAs1DForOutWhenUnconnected=off
  wires:
  MATLAB Function4/1(e_out) -> Err/1
  MATLAB Function2/1(Oy) -> MATLAB Function4/1(Oy)
  Subtract2/1 -> MATLAB Function4/2(e_in)
  MATLAB Function2/2(Ox) -> Subtract2/1
  Act/1 -> MATLAB Function3/1(z)
  Ref/1 -> MATLAB Function2/1(z)
  MATLAB Function3/1(Ox) -> Subtract2/2

== system CombinedExperiment/Simulate Plant Dynamics/x_dot -> x1/Hold this value ==
  In1 : Inport
  Action Port : ActionPort  ActionPortLabel=if(u1 ~= 0)
  Out1 : Outport  VectorParamsAs1DForOutWhenUnconnected=off
  wires:
  In1/1 -> Out1/1

== system CombinedExperiment/Simulate Plant Dynamics/x_dot -> x10/Hold this value ==
  In1 : Inport
  Action Port : ActionPort  ActionPortLabel=if(u1 ~= 0)
  Out1 : Outport  VectorParamsAs1DForOutWhenUnconnected=off
  wires:
  In1/1 -> Out1/1

== system CombinedExperiment/Simulate Plant Dynamics/x_dot -> x11/Hold this value ==
  In1 : Inport
  Action Port : ActionPort  ActionPortLabel=if(u1 ~= 0)
  Out1 : Outport  VectorParamsAs1DForOutWhenUnconnected=off
  wires:
  In1/1 -> Out1/1

== system CombinedExperiment/Simulate Plant Dynamics/x_dot -> x12/Hold this value ==
  In1 : Inport
  Action Port : ActionPort  ActionPortLabel=if(u1 ~= 0)
  Out1 : Outport  VectorParamsAs1DForOutWhenUnconnected=off
  wires:
  In1/1 -> Out1/1

== system CombinedExperiment/Simulate Plant Dynamics/x_dot -> x13/Hold this value ==
  In1 : Inport
  Action Port : ActionPort  ActionPortLabel=if(u1 ~= 0)
  Out1 : Outport  VectorParamsAs1DForOutWhenUnconnected=off
  wires:
  In1/1 -> Out1/1

== system CombinedExperiment/Simulate Plant Dynamics/x_dot -> x14/Hold this value ==
  In1 : Inport
  Action Port : ActionPort  ActionPortLabel=if(u1 ~= 0)
  Out1 : Outport  VectorParamsAs1DForOutWhenUnconnected=off
  wires:
  In1/1 -> Out1/1

== system CombinedExperiment/Simulate Plant Dynamics/x_dot -> x16/Hold this value ==
  In1 : Inport
  Action Port : ActionPort  ActionPortLabel=if(u1 ~= 0)
  Out1 : Outport  VectorParamsAs1DForOutWhenUnconnected=off
  wires:
  In1/1 -> Out1/1

== system CombinedExperiment/Simulate Plant Dynamics/x_dot -> x17/Hold this value ==
  In1 : Inport
  Action Port : ActionPort  ActionPortLabel=if(u1 ~= 0)
  Out1 : Outport  VectorParamsAs1DForOutWhenUnconnected=off
  wires:
  In1/1 -> Out1/1

== system CombinedExperiment/Simulate Plant Dynamics/x_dot -> x2/Hold this value ==
  In1 : Inport
  Action Port : ActionPort  ActionPortLabel=if(u1 ~= 0)
  Out1 : Outport  VectorParamsAs1DForOutWhenUnconnected=off
  wires:
  In1/1 -> Out1/1

== system CombinedExperiment/Simulate Plant Dynamics/x_dot -> x3/Hold this value ==
  In1 : Inport
  Action Port : ActionPort  ActionPortLabel=if(u1 ~= 0)
  Out1 : Outport  VectorParamsAs1DForOutWhenUnconnected=off
  wires:
  In1/1 -> Out1/1

== system CombinedExperiment/Simulate Plant Dynamics/x_dot -> x4/Hold this value ==
  In1 : Inport
  Action Port : ActionPort  ActionPortLabel=if(u1 ~= 0)
  Out1 : Outport  VectorParamsAs1DForOutWhenUnconnected=off
  wires:
  In1/1 -> Out1/1

== system CombinedExperiment/Simulate Plant Dynamics/x_dot -> x5/Hold this value ==
  In1 : Inport
  Action Port : ActionPort  ActionPortLabel=if(u1 ~= 0)
  Out1 : Outport  VectorParamsAs1DForOutWhenUnconnected=off
  wires:
  In1/1 -> Out1/1

== system CombinedExperiment/Simulate Plant Dynamics/x_dot -> x6/Hold this value ==
  In1 : Inport
  Action Port : ActionPort  ActionPortLabel=if(u1 ~= 0)
  Out1 : Outport  VectorParamsAs1DForOutWhenUnconnected=off
  wires:
  In1/1 -> Out1/1

== system CombinedExperiment/Simulate Plant Dynamics/x_dot -> x7/Hold this value ==
  In1 : Inport
  Action Port : ActionPort  ActionPortLabel=if(u1 ~= 0)
  Out1 : Outport  VectorParamsAs1DForOutWhenUnconnected=off
  wires:
  In1/1 -> Out1/1

== system CombinedExperiment/Simulate Plant Dynamics/x_dot -> x8/Hold this value ==
  In1 : Inport
  Action Port : ActionPort  ActionPortLabel=if(u1 ~= 0)
  Out1 : Outport  VectorParamsAs1DForOutWhenUnconnected=off
  wires:
  In1/1 -> Out1/1

== system CombinedExperiment/Simulate Plant Dynamics/x_dot -> x9/Hold this value ==
  In1 : Inport
  Action Port : ActionPort  ActionPortLabel=if(u1 ~= 0)
  Out1 : Outport  VectorParamsAs1DForOutWhenUnconnected=off
  wires:
  In1/1 -> Out1/1

== system CombinedExperiment/From Force//Torque to PWM Signal/Change BLACK Behavior/Calculate Thruster ON//OFF/Rotate Forces to Inertial ==
  "F_b " : Inport
  Rz : Inport  Port=2
  Create Rotation Matrix : MATLAB Function  TreatAsAtomicUnit=on
  Rotate F_b to F_I : Product  Multiplication=Matrix(*)
  F_I : Outport  VectorParamsAs1DForOutWhenUnconnected=off
  wires:
  "F_b "/1 -> Rotate F_b to F_I/2
  Rotate F_b to F_I/1 -> F_I/1
  Create Rotation Matrix/1(C_Ib) -> Rotate F_b to F_I/1
  Rz/1 -> Create Rotation Matrix/1(Rz)

== system CombinedExperiment/From Force//Torque to PWM Signal/Change BLACK Behavior/Calculate Thruster ON//OFF/pseudo-inverse ==
  H : Inport
  Product : Product  Multiplication=Matrix(*)
  Product1 : Product  Inputs=/  Multiplication=Matrix(*)
  Product2 : Product  Multiplication=Matrix(*)
  transpose : PermuteDimensions
  invH : Outport  VectorParamsAs1DForOutWhenUnconnected=off
  wires:
  Product2/1 -> invH/1
  transpose/1 -> Product/2, Product2/1
  Product/1 -> Product1/1
  H/1 -> Product/1, transpose/1
  Product1/1 -> Product2/2

== system CombinedExperiment/From Force//Torque to PWM Signal/Change BLUE Behavior/Calculate Thruster ON//OFF/Rotate Forces to Inertial ==
  "F_b " : Inport
  Rz : Inport  Port=2
  Create Rotation Matrix : MATLAB Function  TreatAsAtomicUnit=on
  Rotate F_b to F_I : Product  Multiplication=Matrix(*)
  F_I : Outport  VectorParamsAs1DForOutWhenUnconnected=off
  wires:
  "F_b "/1 -> Rotate F_b to F_I/2
  Rotate F_b to F_I/1 -> F_I/1
  Create Rotation Matrix/1(C_Ib) -> Rotate F_b to F_I/1
  Rz/1 -> Create Rotation Matrix/1(Rz)

== system CombinedExperiment/From Force//Torque to PWM Signal/Change BLUE Behavior/Calculate Thruster ON//OFF/pseudo-inverse ==
  H : Inport
  Product : Product  Multiplication=Matrix(*)
  Product1 : Product  Inputs=/  Multiplication=Matrix(*)
  Product2 : Product  Multiplication=Matrix(*)
  transpose : PermuteDimensions
  invH : Outport  VectorParamsAs1DForOutWhenUnconnected=off
  wires:
  Product2/1 -> invH/1
  transpose/1 -> Product/2, Product2/1
  Product/1 -> Product1/1
  H/1 -> Product/1, transpose/1
  Product1/1 -> Product2/2

== system CombinedExperiment/From Force//Torque to PWM Signal/Change RED Behavior/Calculate Thruster ON//OFF/Rotate Forces to Inertial ==
  "F_b " : Inport
  Rz : Inport  Port=2
  Create Rotation Matrix : MATLAB Function  TreatAsAtomicUnit=on
  Rotate F_b to F_I : Product  Multiplication=Matrix(*)
  F_I : Outport  VectorParamsAs1DForOutWhenUnconnected=off
  wires:
  "F_b "/1 -> Rotate F_b to F_I/2
  Rotate F_b to F_I/1 -> F_I/1
  Create Rotation Matrix/1(C_Ib) -> Rotate F_b to F_I/1
  Rz/1 -> Create Rotation Matrix/1(Rz)

== system CombinedExperiment/From Force//Torque to PWM Signal/Change RED Behavior/Calculate Thruster ON//OFF/pseudo-inverse ==
  H : Inport
  Product : Product  Multiplication=Matrix(*)
  Product1 : Product  Inputs=/  Multiplication=Matrix(*)
  Product2 : Product  Multiplication=Matrix(*)
  transpose : PermuteDimensions
  invH : Outport  VectorParamsAs1DForOutWhenUnconnected=off
  wires:
  Product2/1 -> invH/1
  transpose/1 -> Product/2, Product2/1
  Product/1 -> Product1/1
  H/1 -> Product/1, transpose/1
  Product1/1 -> Product2/2

== system CombinedExperiment/From Torque, Command RW/Change RED Behavior/Wheel RPM to PWM/Convert Wheel Rate to Motor Rate ==
  Wheel RPM : Inport
  Divide : Product  Inputs=**
  Gearbox Ratio : Constant  Value=3375/64
  Motor RPM : Outport  VectorParamsAs1DForOutWhenUnconnected=off
  wires:
  Gearbox Ratio/1 -> Divide/2
  Divide/1 -> Motor RPM/1
  Wheel RPM/1 -> Divide/1

== system CombinedExperiment/From Torque, Command RW/Change RED Behavior/Wheel RPM to PWM/Delay Bank ==
  Status : Inport
  Delay1 : Delay  DelayLength=1  InitialCondition=0
  Delay2 : Delay  InitialCondition=0
  Delay3 : Delay  DelayLength=4  InitialCondition=0
  Delay4 : Delay  DelayLength=5  InitialCondition=0
  Delay5 : Delay  DelayLength=3  InitialCondition=0
  Mostly zeros? : MinMax  Inputs=6
  StatusVector : Outport  VectorParamsAs1DForOutWhenUnconnected=off
  wires:
  Delay3/1 -> Mostly zeros?/5
  Status/1 -> Delay4/1, Delay3/1, Delay5/1, Delay2/1, Delay1/1, Mostly zeros?/1
  Delay2/1 -> Mostly zeros?/3
  Delay4/1 -> Mostly zeros?/6
  Delay5/1 -> Mostly zeros?/4
  Mostly zeros?/1 -> StatusVector/1
  Delay1/1 -> Mostly zeros?/2

== system CombinedExperiment/From Torque, Command RW/Change RED Behavior/Wheel RPM to PWM/Obtain RW Status ==
  GPIO Read1 : embdlinuxlib/GPIO Read  board=Pi 3 Model B  gpio=24  internalResistor=Off  sampleTime=0.1  direction=Input  blockPlatform=Raspberry Pi
      settings: SourceProductBaseCode=SC_BEAGLEBONE_BLUE,RASPPI
  RW_Status : Outport  VectorParamsAs1DForOutWhenUnconnected=off
  wires:
  GPIO Read1/1 -> RW_Status/1

== system CombinedExperiment/From Torque, Command RW/Change RED Behavior/Wheel RPM to PWM/Send Direction to Motor Controller ==
  WheelDir : Inport
  GPIO Write : embdlinuxlib/GPIO Write  board=Pi 3 Model B  gpio=21  direction=Output  blockPlatform=Raspberry Pi
      settings: SourceProductBaseCode=SC_BEAGLEBONE_BLUE,RASPPI
  wires:
  WheelDir/1 -> GPIO Write/1

== system CombinedExperiment/From Torque, Command RW/Change RED Behavior/Wheel RPM to PWM/Send PWM to Motor Controller ==
  MotorPWM : Inport
  PWM1 : raspberrypiBasiclib/PWM  board=Pi 3 Model B  Pin_=18  Frequency=10  blockPlatform=Raspberry Pi
      settings: SourceProductBaseCode=RASPPI
  wires:
  MotorPWM/1 -> PWM1/1

== system CombinedExperiment/From Torque, Command RW/Change RED Behavior/Wheel RPM to PWM/Turn on Motor ==
  EnableSig : Inport
  GPIO Write1 : embdlinuxlib/GPIO Write  board=Pi 3 Model B  gpio=25  direction=Output  blockPlatform=Raspberry Pi
      settings: SourceProductBaseCode=SC_BEAGLEBONE_BLUE,RASPPI
  wires:
  EnableSig/1 -> GPIO Write1/1

== system CombinedExperiment/Grab PhaseSpace Data via UDP/Use Hardware to Obtain States/Using RED+BLACK, or RED+BLACK+ARM/Is this a simulation? ==
  Constant : Constant  Value=simMode  SampleTime=-1
  isSim : Outport  VectorParamsAs1DForOutWhenUnconnected=off
  wires:
  Constant/1 -> isSim/1
